simulink model "RackAndPinion1"  (R2023a)
settings: Solver=VariableStepAuto  StartTime=0.0  StopTime=10.0  RelTol=1e-3
settings Model: Creator=mrrom  LastModifiedBy=mrrom

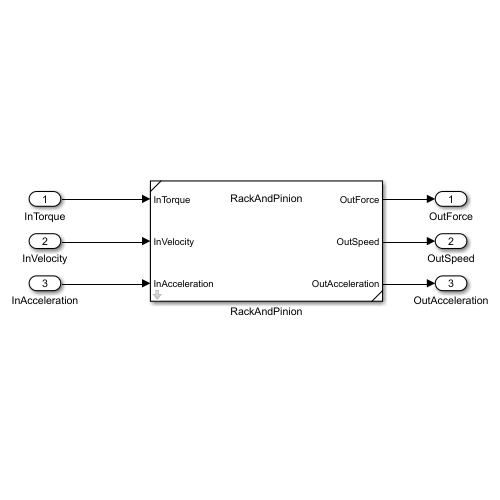
[thumbnail: Simulink's stored preview of the top-level diagram]
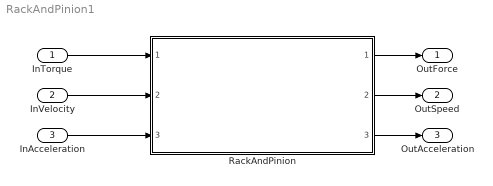
== system RackAndPinion1 ==
  InTorque : Inport
  InVelocity : Inport  Port=2
  InAcceleration : Inport  Port=3
  RackAndPinion : Subsystem  ReferencedSubsystem=RackAndPinion  i_rp=20000  vis_friction_coef_rp=0.002  J_pinion=1e-6
  OutForce : Outport
  OutSpeed : Outport  Port=2
  OutAcceleration : Outport  Port=3
  wires:
  InTorque/1 -> RackAndPinion/1
  InVelocity/1 -> RackAndPinion/2
  InAcceleration/1 -> RackAndPinion/3
  RackAndPinion/1 -> OutForce/1
  RackAndPinion/2 -> OutSpeed/1
  RackAndPinion/3 -> OutAcceleration/1
